simulink subsystem "Motors_ThorneFleissner"  (R2020b)
settings: Solver=VariableStepAuto  StartTime=0.0  StopTime=10.0  RelTol=1e-3
settings Model: Creator=rthom  LastModifiedBy=rthom

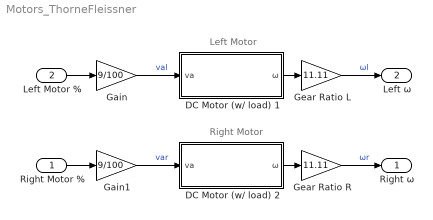
== system Motors_ThorneFleissner ==
  note: Left Motor
  note: Right Motor
  Right Motor % : Inport
  Left Motor % : Inport  Port=2
  DC Motor (w/ load) 1 : Subsystem
  DC Motor (w/ load) 2 : Subsystem
  Gain : Gain  Gain=9/100
  Gain1 : Gain  Gain=9/100
  Gear Ratio L : Gain  Gain=11.11
  Gear Ratio R : Gain  Gain=11.11
  Right ω : Outport
  Left ω : Outport  Port=2
  wires:
  DC Motor (w/ load) 1/1(ω) -> Gear Ratio L/1
  Right Motor %/1 -> Gain1/1
  Gear Ratio L/1 -> Left ω/1  "ωl"
  DC Motor (w/ load) 2/1(ω) -> Gear Ratio R/1
  Left Motor %/1 -> Gain/1
  Gain/1 -> DC Motor (w/ load) 1/1(va)  "val"
  Gear Ratio R/1 -> Right ω/1  "ωr"
  Gain1/1 -> DC Motor (w/ load) 2/1(va)  "var"

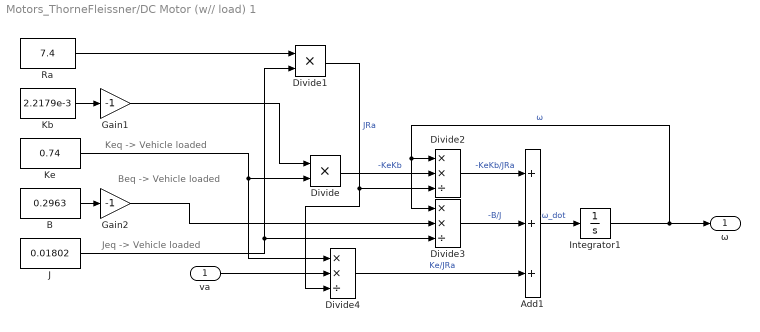
== system Motors_ThorneFleissner/DC Motor (w// load) 1 ==
  note: Beq -> Vehicle loaded
  note: Jeq -> Vehicle loaded
  note: Keq -> Vehicle loaded
  va : Inport
  Add1 : Sum  Inputs=+++
  B : Constant  Value=0.2963
  Divide : Product  Inputs=**
  Divide1 : Product  Inputs=**
  Divide2 : Product  Inputs=**/
  Divide3 : Product  Inputs=**/
  Divide4 : Product  Inputs=**/
  Gain1 : Gain  Gain=-1
  Gain2 : Gain  Gain=-1
  Integrator1 : Integrator
  J : Constant  Value=0.01802
  Kb : Constant  Value=2.2179e-3
  Ke : Constant  Value=0.74
  Ra : Constant  Value=7.4
  ω : Outport
  wires:
  Integrator1/1 -> ω/1, Divide2/1, Divide3/1  "ω"
  Divide4/1 -> Add1/3  "Ke/JRa"
  Divide1/1 -> Divide4/3, Divide2/3  "JRa"
  Divide/1 -> Divide2/2  "-KeKb"
  Gain1/1 -> Divide/1
  va/1 -> Divide4/2
  Add1/1 -> Integrator1/1  "ω_dot"
  Gain2/1 -> Divide3/2
  B/1 -> Gain2/1
  J/1 -> Divide3/3, Divide1/2
  Ke/1 -> Divide/2, Divide4/1
  Kb/1 -> Gain1/1
  Ra/1 -> Divide1/1
  Divide3/1 -> Add1/2  "-B/J"
  Divide2/1 -> Add1/1  "-KeKb/JRa"

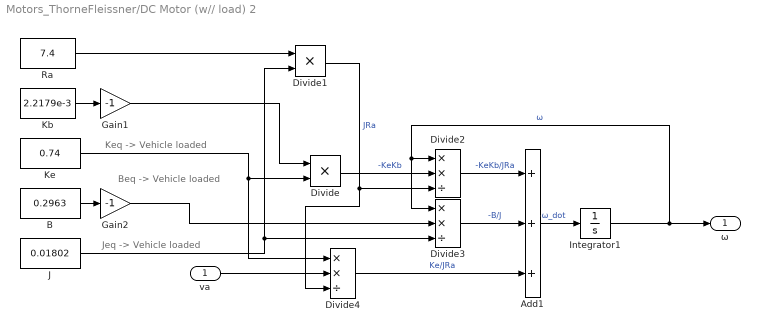
== system Motors_ThorneFleissner/DC Motor (w// load) 2 ==
  note: Beq -> Vehicle loaded
  note: Jeq -> Vehicle loaded
  note: Keq -> Vehicle loaded
  va : Inport
  Add1 : Sum  Inputs=+++
  B : Constant  Value=0.2963
  Divide : Product  Inputs=**
  Divide1 : Product  Inputs=**
  Divide2 : Product  Inputs=**/
  Divide3 : Product  Inputs=**/
  Divide4 : Product  Inputs=**/
  Gain1 : Gain  Gain=-1
  Gain2 : Gain  Gain=-1
  Integrator1 : Integrator
  J : Constant  Value=0.01802
  Kb : Constant  Value=2.2179e-3
  Ke : Constant  Value=0.74
  Ra : Constant  Value=7.4
  ω : Outport
  wires:
  Integrator1/1 -> ω/1, Divide2/1, Divide3/1  "ω"
  Divide4/1 -> Add1/3  "Ke/JRa"
  Divide1/1 -> Divide4/3, Divide2/3  "JRa"
  Divide/1 -> Divide2/2  "-KeKb"
  Gain1/1 -> Divide/1
  va/1 -> Divide4/2
  Add1/1 -> Integrator1/1  "ω_dot"
  Gain2/1 -> Divide3/2
  B/1 -> Gain2/1
  J/1 -> Divide3/3, Divide1/2
  Ke/1 -> Divide/2, Divide4/1
  Kb/1 -> Gain1/1
  Ra/1 -> Divide1/1
  Divide3/1 -> Add1/2  "-B/J"
  Divide2/1 -> Add1/1  "-KeKb/JRa"
